simulink model "F4_Phantom_Prj2_model"  (R2024b)
settings: Solver=VariableStepAuto  StartTime=0.0  StopTime=10.0  RelTol=1e-3
undefined symbols (not defined in the file): InputTime, Kd, Ki, Kp, NewAlt, V_P_1
settings Model: Creator=billy  LastModifiedBy=billy

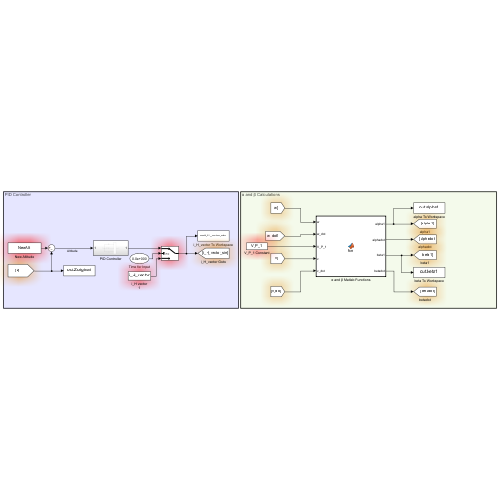
[thumbnail: Simulink's stored preview of the top-level diagram]
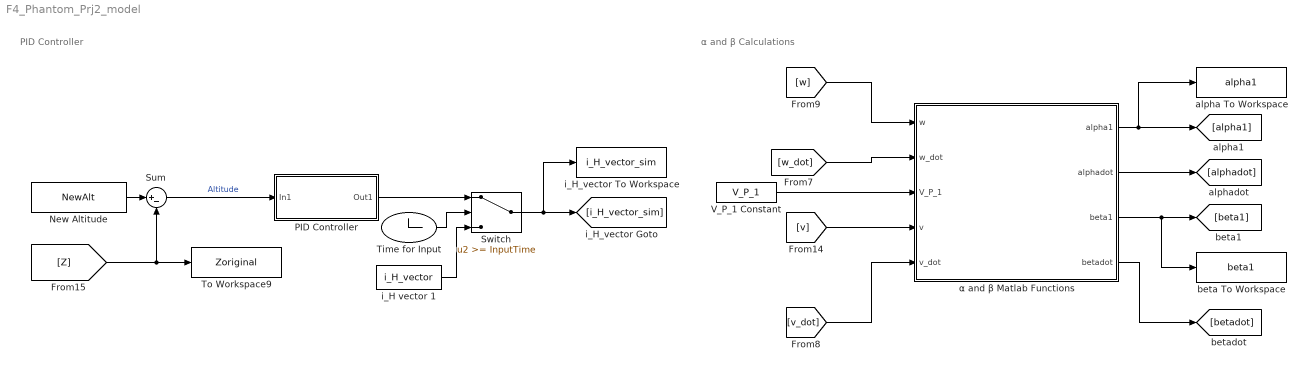
== system F4_Phantom_Prj2_model ==
  note: α and β Calculations
  note: PID Controller
  New Altitude : Constant  Value=NewAlt
  PID Controller : Subsystem
  Sum : Sum  Inputs=|+-
  Switch : Switch  Threshold=InputTime  SaturateOnIntegerOverflow=off  InputSameDT=off
  Time for Input : Clock
      settings: Decimation=1000
  To Workspace9 : ToWorkspace  VariableName=Zoriginal  SaveFormat=Timeseries  SampleTime=-1
  V_P_1 Constant : Constant  Value=V_P_1
  alpha To Workspace : ToWorkspace  VariableName=alpha1  SampleTime=-1
      settings: Save2DSignal=2-D array (concatenate along first dimension)
  beta To Workspace : ToWorkspace  VariableName=beta1  SampleTime=-1
      settings: Save2DSignal=2-D array (concatenate along first dimension)
  i_H vector 1 : FromWorkspace  VariableName=i_H_vector
  i_H_vector To Workspace : ToWorkspace  VariableName=i_H_vector_sim  SampleTime=-1
      settings: Save2DSignal=2-D array (concatenate along first dimension)
  α and β Matlab Functions : MATLAB Function  TreatAsAtomicUnit=on
  wires:
  [Z] -> To Workspace9/1, Sum/2
  i_H vector 1/1 -> Switch/3
  New Altitude/1 -> Sum/1
  Switch/1 -> i_H_vector To Workspace/1, [i_H_vector_sim]
  PID Controller/1(Out1) -> Switch/1
  Sum/1 -> PID Controller/1(In1)  "Altitude"
  Time for Input/1 -> Switch/2
  [v] -> α and β Matlab Functions/4(v)
  [w_dot] -> α and β Matlab Functions/2(w_dot)
  [w] -> α and β Matlab Functions/1(w)
  [v_dot] -> α and β Matlab Functions/5(v_dot)
  α and β Matlab Functions/3(beta1) -> [beta1], beta To Workspace/1
  α and β Matlab Functions/2(alphadot) -> [alphadot]
  α and β Matlab Functions/4(betadot) -> [betadot]
  α and β Matlab Functions/1(alpha1) -> alpha To Workspace/1, [alpha1]
  V_P_1 Constant/1 -> α and β Matlab Functions/3(V_P_1)

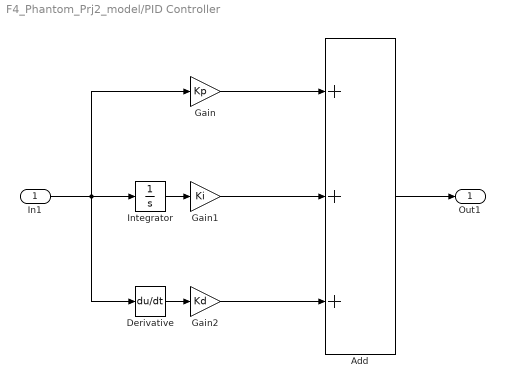
== system F4_Phantom_Prj2_model/PID Controller ==
  In1 : Inport
  Add : Sum  Inputs=+++
  Derivative : Derivative
  Gain : Gain  Gain=Kp
  Gain1 : Gain  Gain=Ki
  Gain2 : Gain  Gain=Kd
  Integrator : Integrator
  Out1 : Outport
  wires:
  In1/1 -> Gain/1, Derivative/1, Integrator/1
  Integrator/1 -> Gain1/1
  Derivative/1 -> Gain2/1
  Gain1/1 -> Add/2
  Gain/1 -> Add/1
  Gain2/1 -> Add/3
  Add/1 -> Out1/1

== matlab function F4_Phantom_Prj2_model/α and β Matlab Functions ==
  data: w input; alpha1 output; alphadot output; beta1 output; w_dot input; V_P_1 input; v input; v_dot input; betadot output
function [alpha1, alphadot, beta1, betadot] = fcn(w, w_dot, V_P_1, v, v_dot)

alpha1 = w/V_P_1;

alphadot = w_dot/V_P_1;

beta1 = v/V_P_1;

betadot = v_dot/V_P_1;
